simulink model "pendulo"  (R2018b)
settings: Solver=ode45  StartTime=0  StopTime=190  MaxStep=.5  RelTol=1e-3  AbsTol=1e-6
libraries: fuzblock x1, simulink x1
settings Model: Creator=Adolfo  LastModifiedBy=Abdullah
settings SolverCC: AutoScaleAbsTol=off
settings DataIOCC: ExternalInput=[]  InitialState=[]  LimitDataPoints=on  MaxDataPoints=10000  SaveFormat=Array  SignalLoggingSaveFormat=ModelDataLogs  SaveOutput=off  SaveTime=off
settings OptimizationCC: BlockReduction=off  BooleanDataType=off  ExpressionDepthLimit=2147483647  InitFltsAndDblsToZero=on  LifeSpan=inf
settings DebuggingCC: SaveWithParameterizedLinksMsg=none  UnderspecifiedInitializationDetection=Classic  MergeDetectMultiDrivingBlocksExec=none  SignalResolutionControl=TryResolveAllWithWarning  MultiTaskDSMMsg=warning  MultiTaskCondExecSysMsg=none  FcnCallInpInsideContextMsg=warning  StateNameClashWarn=warning  SFUnexpectedBacktrackingDiag=warning  SFNoUnconditionalDefaultTransitionDiag=warning  SFExecutionAtInitializationDiag=none
settings HardwareCC: ProdBitPerPointer=32  ProdBitPerSizeT=32  ProdBitPerPtrDiffT=32  ProdLargestAtomicFloat=None  ProdIntDivRoundTo=Undefined  ProdEndianess=Unspecified  ProdWordSize=32  ProdHWDeviceType=32-bit Generic  TargetUnknown=on
settings ModelReferenceCC: PropagateSignalLabelsOutOfModel=off
settings SFSimCC: SimUseLocalCustomCode=off
settings RTWCC: RTWUseLocalCustomCode=off
settings CodeAppCC: StateflowObjectComments=on
settings GRTTargetCC: TargetFcnLib=ansi_tfl_tmw.mat  TargetLangStandard=C89/C90 (ANSI)  CombineOutputUpdateFcns=off  GRTInterface=on
settings ConfigComp: CovMetricSettings=dw  CovHtmlReporting=on  CovSaveCumulativeToWorkspaceVar=on  CovSaveSingleToWorkspaceVar=on  CovExternalEMLEnable=off

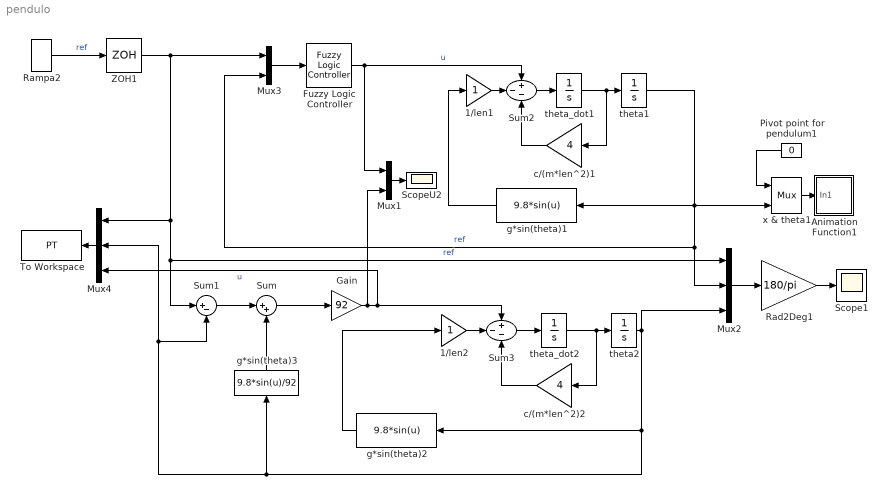
== system pendulo ==
  1/len1 : Gain  SaturateOnIntegerOverflow=on  OutDataTypeStr=Inherit: Same as input  ParamDataTypeStr=Inherit: Same as input
  1/len2 : Gain  SaturateOnIntegerOverflow=on  OutDataTypeStr=Inherit: Same as input  ParamDataTypeStr=Inherit: Same as input
  Animation Function1 : Subsystem  mask(Animation Block){ts=0.05}
      mask prompts: ts "Sample time:"
      mask Display: plot([.1,.9],[.9,.9],[.5,.2],[.9,.25],[.475,.475,.525,.525,.475],[.875,.925,.925,.875,.875])
  Fuzzy Logic Controller : fuzblock/Fuzzy Logic  Controller  FIS="\"neurofuzzy.fis\""  OutputSampleNumber=101  DataType=double  FuzzifiedInputs=off  RuleFiringStrengths=off  RuleOutputs=off  AggregatedOutputs=off  SimulateUsing=Interpreted execution  OutOfRangeInputValueMessage=warning  NoRuleFiredMessage=warning  EmptyOutputFuzzySetMessage=warning
  Gain : Gain  Gain=92
  Mux1 : Mux  Inputs=2
  Mux2 : Mux  Inputs=3
  Mux3 : Mux  Inputs=2
  Mux4 : Mux  Inputs=3
  Pivot point for pendulum1 : Constant  Value=0
  Rad2Deg1 : Gain  Gain=180/pi  SaturateOnIntegerOverflow=on  OutDataTypeStr=Inherit: Same as input  ParamDataTypeStr=Inherit: Same as input
  Rampa2 : simulink/Sources/Ramp  slope=pi/90  start=0  InitialOutput=-pi
  Scope1 : Scope
  ScopeU2 : Scope
  Sum : Sum  Inputs=|++
  Sum1 : Sum  Inputs=|+-
  Sum2 : Sum  Inputs=+--  SaturateOnIntegerOverflow=on  InputSameDT=on  OutDataTypeStr=Inherit: Same as first input
  Sum3 : Sum  Inputs=+--  SaturateOnIntegerOverflow=on  InputSameDT=on  OutDataTypeStr=Inherit: Same as first input
  To Workspace : ToWorkspace  VariableName=PT  SampleTime=-1
  ZOH1 : ZeroOrderHold  SampleTime=10
  c/(m*len^2)1 : Gain  Gain=4  SaturateOnIntegerOverflow=on  OutDataTypeStr=Inherit: Same as input  ParamDataTypeStr=Inherit: Same as input
  c/(m*len^2)2 : Gain  Gain=4  SaturateOnIntegerOverflow=on  OutDataTypeStr=Inherit: Same as input  ParamDataTypeStr=Inherit: Same as input
  g*sin(theta)1 : Fcn  Expr=9.8*sin(u)
  g*sin(theta)2 : Fcn  Expr=9.8*sin(u)
  g*sin(theta)3 : Fcn  Expr=9.8*sin(u)/92
  theta1 : Integrator  InitialCondition=pi  UpperSaturationLimit=200  LowerSaturationLimit=-200
  theta2 : Integrator  InitialCondition=pi  UpperSaturationLimit=200  LowerSaturationLimit=-200
  theta_dot1 : Integrator  InitialCondition=-.1  UpperSaturationLimit=200  LowerSaturationLimit=-200
  theta_dot2 : Integrator  InitialCondition=-.1  UpperSaturationLimit=200  LowerSaturationLimit=-200
  x & theta1 : Mux  Inputs=2
  wires:
  Sum/1 -> Gain/1
  c/(m*len^2)2/1 -> Sum3/3
  theta1/1 -> Mux2/2, Mux3/2, x & theta1/2, g*sin(theta)1/1  "ref"
  g*sin(theta)2/1 -> 1/len2/1
  Fuzzy Logic Controller/1 -> Mux1/1, Sum2/1  "u"
  theta_dot2/1 -> theta2/1, c/(m*len^2)2/1
  1/len1/1 -> Sum2/2
  Pivot point for pendulum1/1 -> x & theta1/1
  1/len2/1 -> Sum3/2
  Sum2/1 -> theta_dot1/1
  ZOH1/1 -> Sum1/1, Mux2/1, Mux4/1, Mux3/1  "ref"
  Mux2/1 -> Rad2Deg1/1
  Rad2Deg1/1 -> Scope1/1
  Sum3/1 -> theta_dot2/1
  theta_dot1/1 -> theta1/1, c/(m*len^2)1/1
  g*sin(theta)1/1 -> 1/len1/1
  x & theta1/1 -> Animation Function1/1(In1)
  c/(m*len^2)1/1 -> Sum2/3
  Gain/1 -> Mux1/2, Sum3/1, Mux4/3  "u"
  Mux3/1 -> Fuzzy Logic Controller/1
  Rampa2/1 -> ZOH1/1  "ref"
  g*sin(theta)3/1 -> Sum/2
  Sum1/1 -> Sum/1
  theta2/1 -> Sum1/2, Mux4/2, g*sin(theta)3/1, g*sin(theta)2/1, Mux2/3
  Mux4/1 -> To Workspace/1
  Mux1/1 -> ScopeU2/1

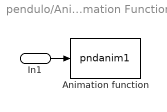
== system pendulo/Animation Function1 ==
  In1 : Inport
  Animation function : S-Function  FunctionName=pndanim1  Parameters=ts  SFunctionDeploymentMode=off  EnableBusSupport=off
      settings: DeleteFcn=if ~isempty(findobj('type','figure','name','simppend Animation'));close('simppend Animation'); end;
  wires:
  In1/1 -> Animation function/1
